simulink model "AGTF30SysLin_PExPIn"  (R2021b)
settings: Solver=ode4  StartTime=0.0  StopTime=2*MWS.In.Ts; %0  FixedStep=MWS.In.Ts  RelTol=1e-3  EnableMultiTasking=on
model workspace: external: MAT-File (data not in the file)
values from neighbouring files (symbols this model uses):
  MWS = setup_initialize(MWS,startPt,SSsolverSP)    [Setup_Simulation.m]    (also in run_AGTF30e_script.m = Setup_Simulation(inputMethod,MWS.In,filename,Mdl,SSsolverSP,)
libraries: Lib_Solve_IterNRSolverJC_TMATS x1
settings Model: Creator=jwchapm2  LastModifiedBy=jlkratz
settings SolverCC: AlgebraicLoopSolver=TrustRegion
settings DataIOCC: LimitDataPoints=on  SaveFormat=Array  ReturnWorkspaceOutputs=off
settings OptimizationCC: LifeSpan=inf
settings DebuggingCC: SFUnexpectedBacktrackingDiag=warning  SFNoUnconditionalDefaultTransitionDiag=warning  SFExecutionAtInitializationDiag=none  SFMachineParentedDataDiag=warning  ArithmeticOperatorsInVariantConditions=warning
settings HardwareCC: ProdBitPerPointer=32  ProdBitPerSizeT=32  ProdBitPerPtrDiffT=32  ProdLargestAtomicFloat=None  ProdIntDivRoundTo=Undefined  ProdEndianess=Unspecified  ProdWordSize=32  ProdHWDeviceType=32-bit Generic
settings ModelReferenceCC: PropagateSignalLabelsOutOfModel=off
settings SFSimCC: SimUseLocalCustomCode=off  CustomCodeUndefinedFunction=UseInterfaceOnly
settings RTWCC: RTWUseLocalCustomCode=off
settings CodeAppCC: StateflowObjectComments=on
settings GRTTargetCC: TargetLangStandard=C89/C90 (ANSI)
settings ConfigComp: CovMetricSettings=dw  CovSaveCumulativeToWorkspaceVar=on  CovSaveSingleToWorkspaceVar=on  CovExternalEMLEnable=off

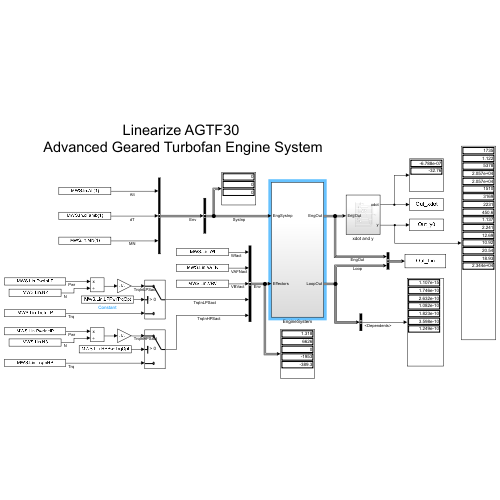
[thumbnail: Simulink's stored preview of the top-level diagram]
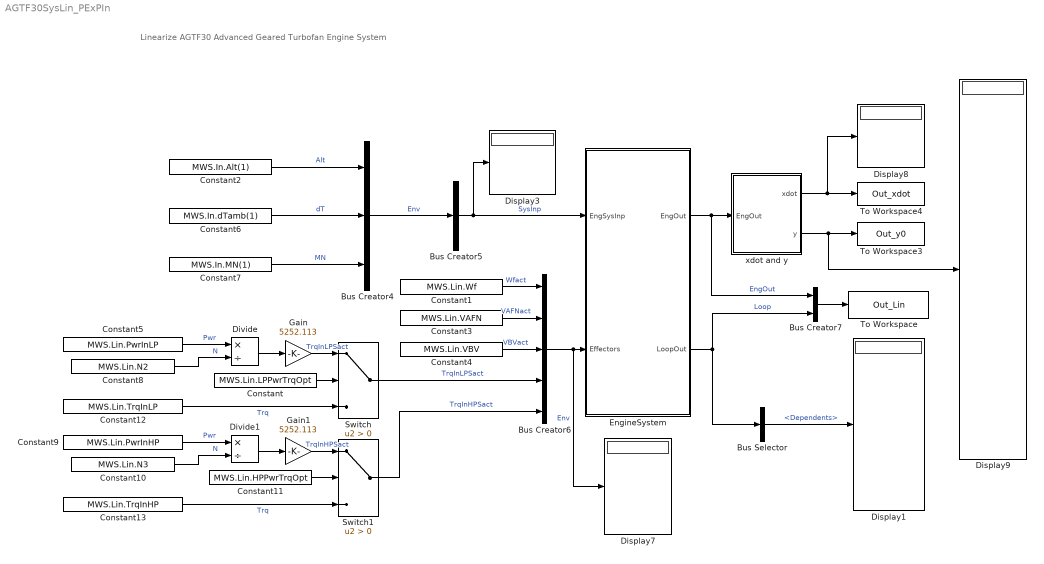
== system AGTF30SysLin_PExPIn ==
  note: Linearize AGTF30
      | Advanced Geared Turbofan Engine System
  Bus Creator4 : BusCreator  Inputs=3
  Bus Creator5 : BusCreator  Inputs=1
  Bus Creator6 : BusCreator  Inputs=5
  Bus Creator7 : BusCreator  Inputs=2
  Bus Selector : BusSelector  OutputSignals=Solver.Dependents
  Constant : Constant  Value=MWS.Lin.LPPwrTrqOpt
  Constant1 : Constant  Value=MWS.Lin.Wf
  Constant10 : Constant  Value=MWS.Lin.N3
  Constant11 : Constant  Value=MWS.Lin.HPPwrTrqOpt
  Constant12 : Constant  Value=MWS.Lin.TrqInLP
  Constant13 : Constant  Value=MWS.Lin.TrqInHP
  Constant2 : Constant  Value=MWS.In.Alt(1)
  Constant3 : Constant  Value=MWS.Lin.VAFN
  Constant4 : Constant  Value=MWS.Lin.VBV
  Constant5 : Constant  Value=MWS.Lin.PwrInLP
  Constant6 : Constant  Value=MWS.In.dTamb(1)
  Constant7 : Constant  Value=MWS.In.MN(1)
  Constant8 : Constant  Value=MWS.Lin.N2
  Constant9 : Constant  Value=MWS.Lin.PwrInHP
  Display{1,3,7..9} (5 alike) : Display
  Divide : Product  Inputs=*/
  Divide1 : Product  Inputs=*/
  EngineSystem : Subsystem
  Gain : Gain  Gain=5252.113
  Gain1 : Gain  Gain=5252.113
  Switch : Switch  Criteria=u2 > Threshold
  Switch1 : Switch  Criteria=u2 > Threshold
  To Workspace : ToWorkspace  VariableName=Out_Lin  SaveFormat=Timeseries  SampleTime=-1
  To Workspace3 : ToWorkspace  VariableName=Out_y0  SaveFormat=Timeseries  SampleTime=-1
  To Workspace4 : ToWorkspace  VariableName=Out_xdot  SaveFormat=Timeseries  SampleTime=-1
  xdot and y : Subsystem
  wires:
  EngineSystem/2(LoopOut) -> Bus Selector/1, Bus Creator7/2  "Loop"
  Bus Creator4/1 -> Bus Creator5/1  "Env"
  Constant6/1 -> Bus Creator4/2  "dT"
  Constant2/1 -> Bus Creator4/1  "Alt"
  Constant7/1 -> Bus Creator4/3  "MN"
  Bus Creator5/1 -> EngineSystem/1(EngSysInp), Display3/1  "SysInp"
  Bus Creator6/1 -> Display7/1, EngineSystem/2(Effectors)  "Env"
  Constant1/1 -> Bus Creator6/1  "Wfact"
  Constant3/1 -> Bus Creator6/2  "VAFNact"
  Constant4/1 -> Bus Creator6/3  "VBVact"
  Constant8/1 -> Divide/2  "N"
  Constant5/1 -> Divide/1  "Pwr"
  Divide/1 -> Gain/1
  Switch/1 -> Bus Creator6/4  "TrqInLPSact"
  Divide1/1 -> Gain1/1
  Constant10/1 -> Divide1/2  "N"
  Constant9/1 -> Divide1/1  "Pwr"
  Switch1/1 -> Bus Creator6/5  "TrqInHPSact"
  EngineSystem/1(EngOut) -> Bus Creator7/1, xdot and y/1(EngOut)  "EngOut"
  xdot and y/1(xdot) -> Display8/1, To Workspace4/1
  xdot and y/2(y) -> Display9/1, To Workspace3/1
  Bus Creator7/1 -> To Workspace/1
  Bus Selector/1 -> Display1/1  "<Dependents>"
  Gain/1 -> Switch/1  "TrqInLPSact"
  Constant/1 -> Switch/2
  Constant11/1 -> Switch1/2
  Gain1/1 -> Switch1/1  "TrqInHPSact"
  Constant12/1 -> Switch/3  "Trq"
  Constant13/1 -> Switch1/3  "Trq"

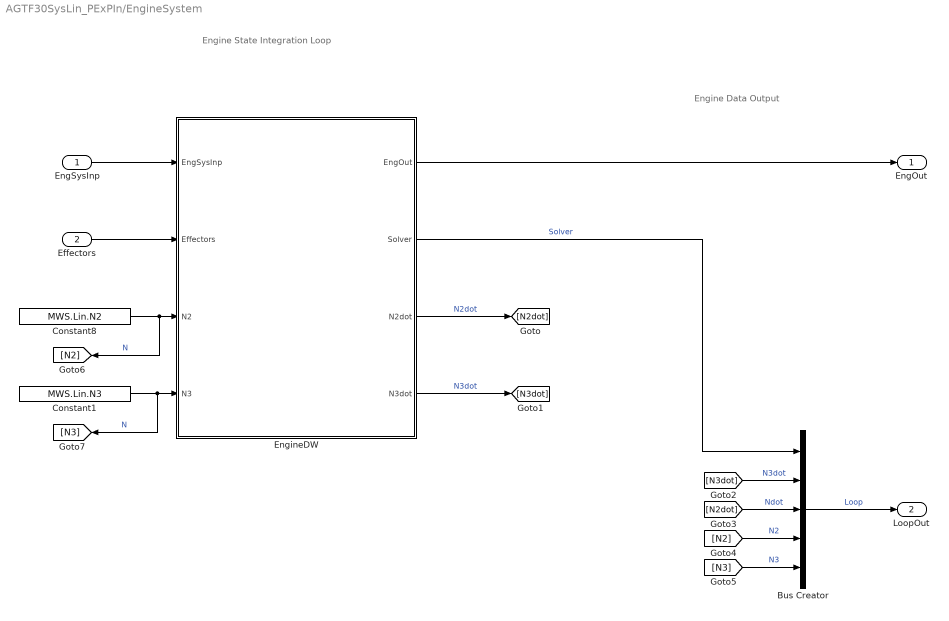
== system AGTF30SysLin_PExPIn/EngineSystem ==
  note: Engine State
      | Integration Loop
  note: Engine Data Output
  EngSysInp : Inport
  Effectors : Inport  Port=2
  Bus Creator : BusCreator  Inputs=5
  Constant1 : Constant  Value=MWS.Lin.N3
  Constant8 : Constant  Value=MWS.Lin.N2
  EngineDW : Subsystem
  EngOut : Outport
  LoopOut : Outport  Port=2
  wires:
  EngSysInp/1 -> EngineDW/1(EngSysInp)
  Effectors/1 -> EngineDW/2(Effectors)
  EngineDW/3(N2dot) -> [N2dot]  "N2dot"
  EngineDW/2(Solver) -> Bus Creator/1  "Solver"
  EngineDW/1(EngOut) -> EngOut/1
  EngineDW/4(N3dot) -> [N3dot]  "N3dot"
  Bus Creator/1 -> LoopOut/1  "Loop"
  [N3dot] -> Bus Creator/2  "N3dot"
  [N2dot] -> Bus Creator/3  "Ndot"
  [N2] -> Bus Creator/4  "N2"
  [N3] -> Bus Creator/5  "N3"
  Constant8/1 -> [N2], EngineDW/3(N2)  "N"
  Constant1/1 -> [N3], EngineDW/4(N3)  "N"

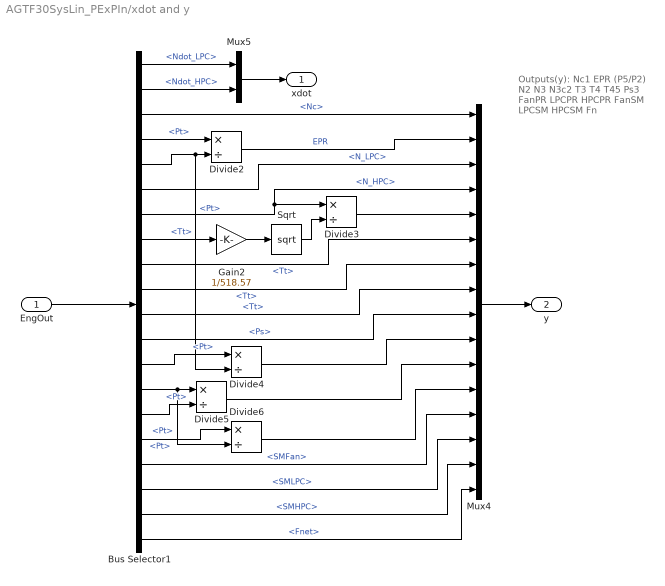
== system AGTF30SysLin_PExPIn/xdot and y ==
  note: Outputs(y):
      | Nc1
      | EPR (P5/P2)
      | N2
      | N3
      | N3c2
      | T3
      | T4
      | T45
      | Ps3
      | FanPR
      | LPCPR
      | HPCPR
      | FanSM
      | LPCSM
      | HPCSM
      | Fn
  EngOut : Inport
  Bus Selector1 : BusSelector  OutputSignals=Shaft.Ndot_LPC,Shaft.Ndot_HPC,Data.FAN_Data.Nc,S5.Pt,S2.Pt,Shaft.N_LPC,Shaft.N_HPC,S2.Tt,S36.Tt,S4.Tt,S45.Tt,S36.Ps,S13.Pt,S25.Pt,S23.Pt,S36.Pt,SM.SMFan,SM.SMLPC,SM.SMHPC,Perf.Fnet
  Divide{2..6} (5 alike) : Product  Inputs=*/
  Gain2 : Gain  Gain=1/518.57
  Mux4 : Mux  Inputs=16
  Mux5 : Mux  Inputs=2
  Sqrt : Sqrt  SaturateOnIntegerOverflow=on
  xdot : Outport
  y : Outport  Port=2
  wires:
  Bus Selector1/6 -> Mux4/3  "<N_LPC>"
  Divide5/1 -> Mux4/11
  Bus Selector1/7 -> Divide3/1, Mux4/4  "<N_HPC>"
  Bus Selector1/9 -> Mux4/6  "<Tt>"
  Bus Selector1/15 -> Divide5/2  "<Pt>"
  Bus Selector1/1 -> Mux5/1  "<Ndot_LPC>"
  Divide2/1 -> Mux4/2  "EPR"
  Bus Selector1/3 -> Mux4/1  "<Nc>"
  Divide4/1 -> Mux4/10
  Divide3/1 -> Mux4/5
  Mux5/1 -> xdot/1
  Gain2/1 -> Sqrt/1
  Divide6/1 -> Mux4/12
  Bus Selector1/18 -> Mux4/14  "<SMLPC>"
  Bus Selector1/10 -> Mux4/7  "<Tt>"
  Bus Selector1/11 -> Mux4/8  "<Tt>"
  Bus Selector1/12 -> Mux4/9  "<Ps>"
  Bus Selector1/17 -> Mux4/13  "<SMFan>"
  Bus Selector1/2 -> Mux5/2  "<Ndot_HPC>"
  Bus Selector1/14 -> Divide6/2, Divide5/1  "<Pt>"
  Bus Selector1/4 -> Divide2/1  "<Pt>"
  Bus Selector1/8 -> Gain2/1  "<Tt>"
  Bus Selector1/20 -> Mux4/16  "<Fnet>"
  Sqrt/1 -> Divide3/2
  Bus Selector1/13 -> Divide4/1  "<Pt>"
  Bus Selector1/5 -> Divide4/2, Divide2/2  "<Pt>"
  Bus Selector1/19 -> Mux4/15  "<SMHPC>"
  Bus Selector1/16 -> Divide6/1  "<Pt>"
  EngOut/1 -> Bus Selector1/1
  Mux4/1 -> y/1

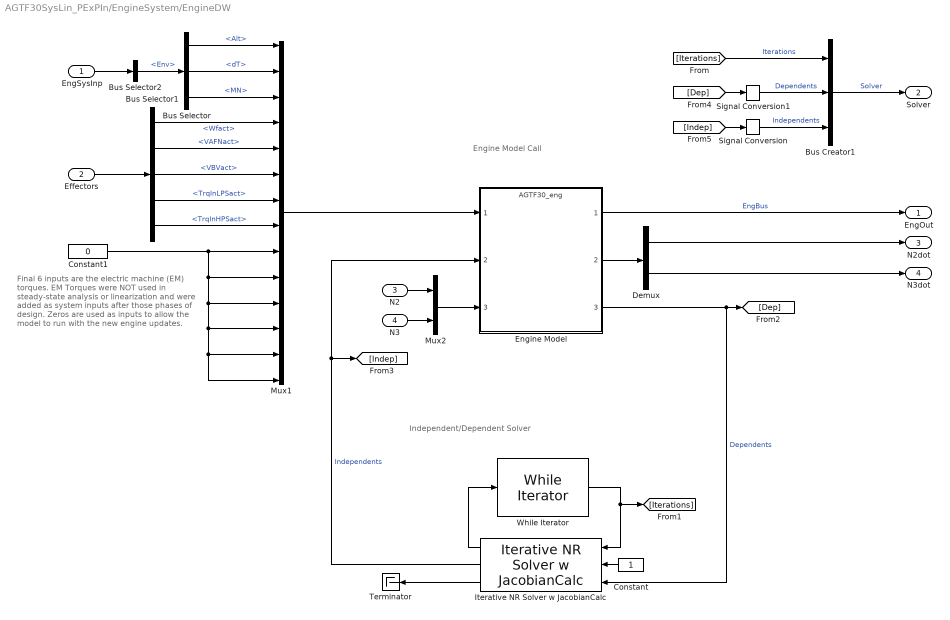
== system AGTF30SysLin_PExPIn/EngineSystem/EngineDW ==
  note: Independent/Dependent Solver
  note: Engine Model Call
  note: Final 6 inputs are the electric machine
      | (EM) torques. EM Torques were NOT used
      | in steady-state analysis or linearization and
      | were added as system inputs after those
      | phases of design. Zeros are used as inputs
      | to allow the model to run with the new engine
      | updates.
  EngSysInp : Inport
  Effectors : Inport  Port=2
  N2 : Inport  Port=3
  N3 : Inport  Port=4
  Bus Creator1 : BusCreator  Inputs=3
  Bus Selector : BusSelector  OutputSignals=Alt,dT,MN
  Bus Selector1 : BusSelector  OutputSignals=Wfact,VAFNact,VBVact,TrqInLPSact,TrqInHPSact
  Bus Selector2 : BusSelector  OutputSignals=Env
  Constant : Constant
  Constant1 : Constant  Value=0
  Demux : Demux  Outputs=2
  Engine Model : ModelReference  ModelNameDialog=AGTF30_eng.mdl  SimulationMode=Normal  ModelReferenceVersion=14.9
  Iterative NR Solver w JacobianCalc : Lib_Solve_IterNRSolverJC_TMATS/Iterative NR Solver w JacobianCalc  SJac_Per_M=MWS.Init.Solver.Dyn.JPer  SNR_IC_M=MWS.Init.Solver.Dyn.IC  SNR_DX_M=MWS.Init.Solver.Dyn.dX  SNR_Mx_M=100000  SNR_Mn_M=0.0001  SJacobianAttempts_M=MWS.Init.Solver.Dyn.NRA  Cond_Limits_M=MWS.Init.Solver.Dyn.Lim
  Mux1 : Mux  Inputs=14
  Mux2 : Mux  Inputs=2
  Signal Conversion : SignalConversion  OverrideOpt=off
  Signal Conversion1 : SignalConversion  OverrideOpt=off
  Terminator : Terminator
  While Iterator : WhileIterator  MaxIters=MWS.Init.Solver.Dyn.Max_Iter  WhileBlockType=do-while  ShowIterationPort=on
  EngOut : Outport
  Solver : Outport  Port=2
  N2dot : Outport  Port=3
  N3dot : Outport  Port=4
  wires:
  Engine Model/1 -> EngOut/1  "EngBus"
  Mux1/1 -> Engine Model/1
  EngSysInp/1 -> Bus Selector2/1
  Effectors/1 -> Bus Selector1/1
  Constant/1 -> Iterative NR Solver w JacobianCalc/2
  Iterative NR Solver w JacobianCalc/2 -> Engine Model/2, [Indep]  "Independents"
  Engine Model/3 -> Iterative NR Solver w JacobianCalc/3, [Dep]  "Dependents"
  While Iterator/1 -> [Iterations], Iterative NR Solver w JacobianCalc/1
  Iterative NR Solver w JacobianCalc/1 -> While Iterator/1
  Engine Model/2 -> Demux/1
  Mux2/1 -> Engine Model/3
  Iterative NR Solver w JacobianCalc/3 -> Terminator/1
  N2/1 -> Mux2/1
  N3/1 -> Mux2/2
  Demux/1 -> N2dot/1
  Demux/2 -> N3dot/1
  Bus Selector/1 -> Mux1/1  "<Alt>"
  Bus Selector/2 -> Mux1/2  "<dT>"
  Bus Selector/3 -> Mux1/3  "<MN>"
  Bus Selector1/3 -> Mux1/6  "<VBVact>"
  Bus Selector1/1 -> Mux1/4  "<Wfact>"
  [Iterations] -> Bus Creator1/1  "Iterations"
  Bus Creator1/1 -> Solver/1  "Solver"
  [Dep] -> Signal Conversion1/1
  [Indep] -> Signal Conversion/1
  Signal Conversion/1 -> Bus Creator1/3  "Independents"
  Signal Conversion1/1 -> Bus Creator1/2  "Dependents"
  Bus Selector1/2 -> Mux1/5  "<VAFNact>"
  Bus Selector2/1 -> Bus Selector/1  "<Env>"
  Bus Selector1/4 -> Mux1/7  "<TrqInLPSact>"
  Bus Selector1/5 -> Mux1/8  "<TrqInHPSact>"
  Constant1/1 -> Mux1/14, Mux1/13, Mux1/12, Mux1/11, Mux1/10, Mux1/9
